simulink model "Clutch_LookUp_Model"  (R2020a)
settings: Solver=VariableStepAuto  StartTime=0.0  StopTime=10.0  RelTol=1e-3
values from neighbouring files (symbols this model uses):
  be = 2.0    [DictionaryclutchParamters.sldd]
  bv = 1.0    [DictionaryclutchParamters.sldd]
  Ie = 1.0    [DictionaryclutchParamters.sldd]
  Iv = 5.0    [DictionaryclutchParamters.sldd]
  muk = 1.0    [DictionaryclutchParamters.sldd]
  mus = 1.5    [DictionaryclutchParamters.sldd]
  R = 1.0    [DictionaryclutchParamters.sldd]
settings Model: DataDictionary=DictionaryclutchParamters.sldd  Creator=DELL  LastModifiedBy=DELL

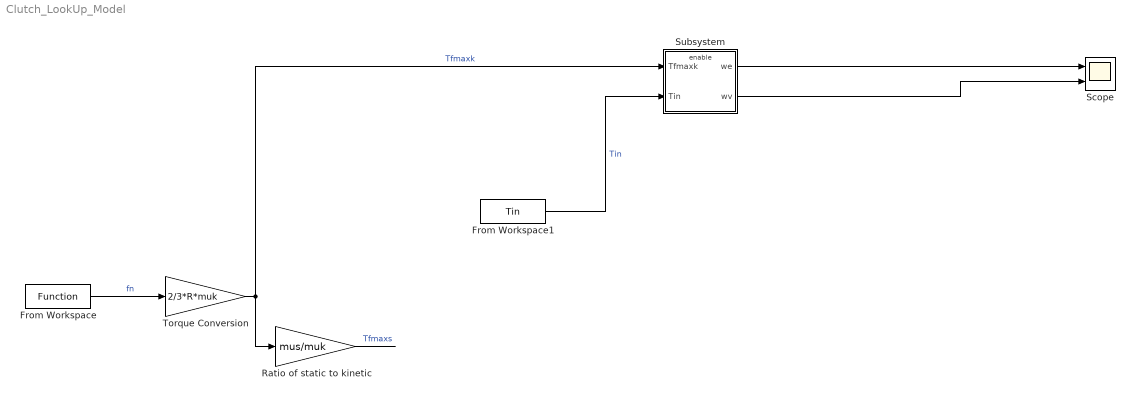
== system Clutch_LookUp_Model ==
  From Workspace : FromWorkspace  VariableName=Function
  From Workspace1 : FromWorkspace  VariableName=Tin
  Ratio of static to kinetic : Gain  Gain=mus/muk  SaturateOnIntegerOverflow=on  OutDataTypeStr=Inherit: Same as input  ParamDataTypeStr=Inherit: Same as input
  Scope : Scope  NumInputPorts=2
  Subsystem : Subsystem
  Torque Conversion : Gain  Gain=2/3*R*muk  SaturateOnIntegerOverflow=on  OutDataTypeStr=Inherit: Same as input  ParamDataTypeStr=Inherit: Same as input
  wires:
  Ratio of static to kinetic/1 -> ?  "Tfmaxs"
  Torque Conversion/1 -> Subsystem/1(Tfmaxk), Ratio of static to kinetic/1  "Tfmaxk"
  From Workspace/1 -> Torque Conversion/1  "fn"
  From Workspace1/1 -> Subsystem/2(Tin)  "Tin"
  Subsystem/1(we) -> Scope/1
  Subsystem/2(wv) -> Scope/2

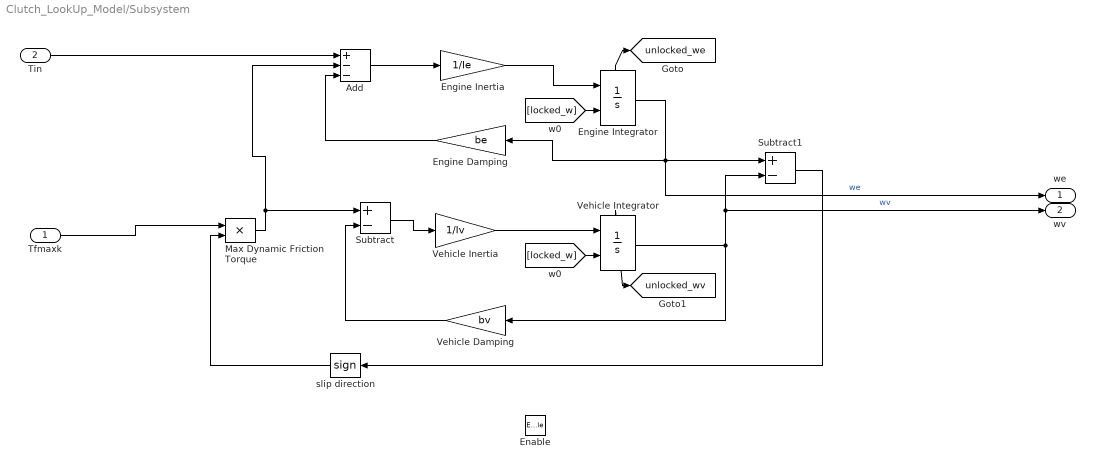
== system Clutch_LookUp_Model/Subsystem ==
  Tfmaxk : Inport
  Tin : Inport  Port=2
  Enable : EnablePort  StatesWhenEnabling=reset
  Add : Sum  Inputs=+--
  Engine Damping : Gain  Gain=be  SaturateOnIntegerOverflow=on  OutDataTypeStr=Inherit: Same as input  ParamDataTypeStr=Inherit: Same as input
  Engine Inertia : Gain  Gain=1/Ie  SaturateOnIntegerOverflow=on  OutDataTypeStr=Inherit: Same as input  ParamDataTypeStr=Inherit: Same as input
  Engine Integrator : Integrator  InitialConditionSource=external  ShowStatePort=on
  Max Dynamic Friction Torque : Product  InputSameDT=on  RndMeth=Zero  SaturateOnIntegerOverflow=on  OutDataTypeStr=Inherit: Same as first input
  Subtract : Sum  Inputs=+-
  Subtract1 : Sum  Inputs=+-
  Vehicle Damping : Gain  Gain=bv  SaturateOnIntegerOverflow=on  OutDataTypeStr=Inherit: Same as input  ParamDataTypeStr=Inherit: Same as input
  Vehicle Inertia : Gain  Gain=1/Iv  SaturateOnIntegerOverflow=on  OutDataTypeStr=Inherit: Same as input  ParamDataTypeStr=Inherit: Same as input
  Vehicle Integrator : Integrator  InitialConditionSource=external  ShowStatePort=on
  slip direction : Signum
  we : Outport
  wv : Outport  Port=2
  tag scope: unlocked_we=global, unlocked_wv=global
  wires:
  Engine Inertia/1 -> Engine Integrator/1
  [locked_w] -> Vehicle Integrator/2
  Engine Damping/1 -> Add/3
  Max Dynamic Friction Torque/1 -> Add/2, Subtract/1
  Tin/1 -> Add/1
  Vehicle Inertia/1 -> Vehicle Integrator/1
  Vehicle Integrator/1 -> wv/1, Subtract1/2, Vehicle Damping/1  "wv"
  Add/1 -> Engine Inertia/1
  Engine Integrator/State -> [unlocked_we]
  [locked_w] -> Engine Integrator/2
  slip direction/1 -> Max Dynamic Friction Torque/2
  Vehicle Integrator/State -> [unlocked_wv]
  Vehicle Damping/1 -> Subtract/2
  Engine Integrator/1 -> we/1, Engine Damping/1, Subtract1/1  "we"
  Subtract/1 -> Vehicle Inertia/1
  Subtract1/1 -> slip direction/1
  Tfmaxk/1 -> Max Dynamic Friction Torque/1
